simulink model "Q2sim5"  (R2022a)
settings: Solver=VariableStepAuto  StartTime=0.0  StopTime=50  FixedStep=1e-4  RelTol=1e-3
values from neighbouring files (symbols this model uses):
  A = [0 1  0              0 ... (first row only)    [Q2.m]
  Ams = Ms    [Q2.m]
  B = [0; 1/M; 0; -1/(M*L)]    [Q2.m]
  Bms = Ns    [Q2.m]
  C = [1 0 0 0]    [Q2.m]
  Dsim = zeros(4,1)    [Q2.m]
  Kms = Kas(5:7)    [Q2.m]
  Ks = Kas (1:4)    [Q2.m]
  x0 = [0 0 deg2rad(51) 0]    [Q2.m]
settings Model: Creator=Crippa  LastModifiedBy=Crippa
settings SolverCC: ZeroCrossControl=DisableAll

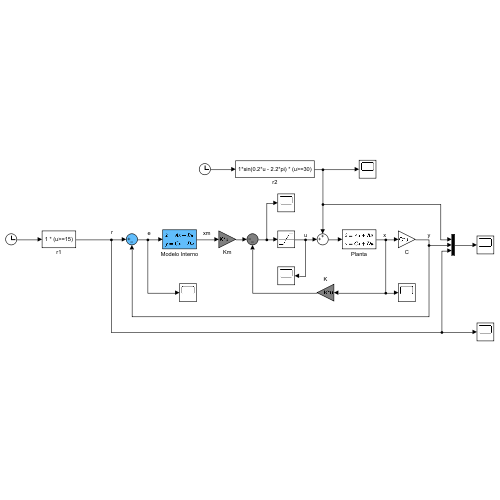
[thumbnail: Simulink's stored preview of the top-level diagram]
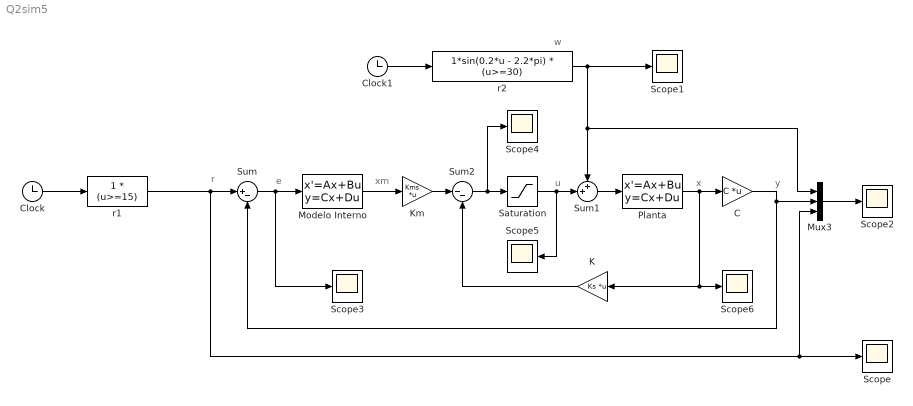
== system Q2sim5 ==
  note: xm
  note: r
  note: x
  note: u
  note: e
  note: y
  note: w
  C : Gain  Gain=C  Multiplication=Matrix(K*u)
  Clock : Clock
  Clock1 : Clock
  K : Gain  Gain=Ks  Multiplication=Matrix(K*u)
  Km : Gain  Gain=Kms  Multiplication=Matrix(K*u)
  Modelo Interno : StateSpace  A=Ams  B=Bms  C=eye(3)  D=zeros(3,1)  InitialCondition=0  ParameterTunability=Optimized
  Mux3 : Mux  Inputs=3
  Planta : StateSpace  A=A  B=B  C=eye(4)  D=Dsim  InitialCondition=x0
  Saturation : Saturate  UpperLimit=150  LowerLimit=-150
  Scope{,1..6} (7 alike) : Scope
  Sum : Sum  Inputs=|+-
  Sum1 : Sum  Inputs=++|
  Sum2 : Sum  Inputs=|--
  r1 : Fcn  Expr=1 * (u>=15)
  r2 : Fcn  Expr=1*sin(0.2*u - 2.2*pi) * (u>=30)
  wires:
  K/1 -> Sum2/2
  Modelo Interno/1 -> Km/1
  r1/1 -> Sum/1, Scope/1, Mux3/3
  Km/1 -> Sum2/1
  Sum2/1 -> Saturation/1, Scope4/1
  Clock/1 -> r1/1
  Mux3/1 -> Scope2/1
  Sum/1 -> Modelo Interno/1, Scope3/1
  Planta/1 -> C/1, Scope6/1, K/1
  C/1 -> Mux3/2, Sum/2
  r2/1 -> Scope1/1, Sum1/1, Mux3/1
  Saturation/1 -> Sum1/2, Scope5/1
  Sum1/1 -> Planta/1
  Clock1/1 -> r2/1
